simulink model "Backstep"  (Simulink 7.0)
settings: Solver=ode45  StartTime=0.0  StopTime=1000.0  RelTol=1e-3
undefined symbols (not defined in the file or in its folder): C_calc
libraries: marine_gnc x3, fordypningsprosjekt x1, simulink x1
settings Model: Creator=anderga  LastModifiedBy=anderga

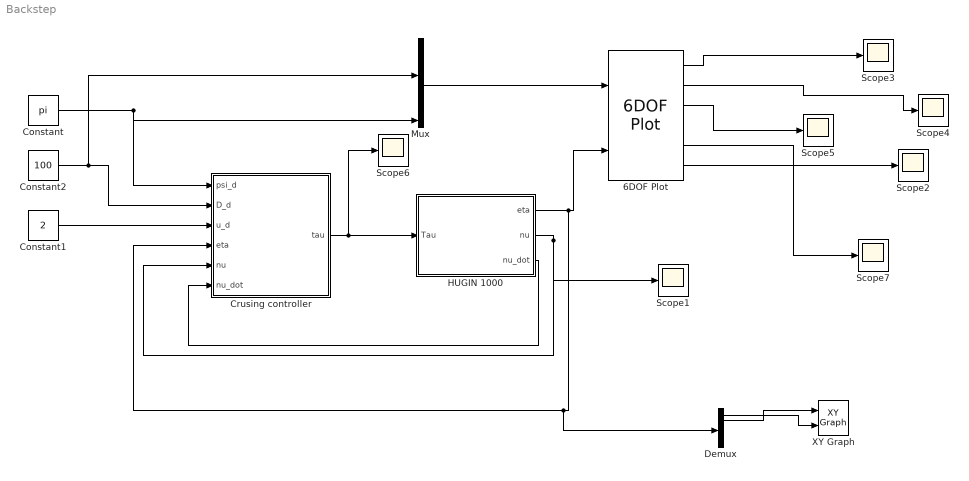
== system Backstep ==
  6DOF Plot : fordypningsprosjekt/6DOF Plot  SystemSampleTime=-1
  Constant : Constant  Value=pi  OutDataType=sfix(16)  OutScaling=2^0
  Constant1 : Constant  Value=2  OutDataType=sfix(16)  OutScaling=2^0
  Constant2 : Constant  Value=100  OutDataType=sfix(16)  OutScaling=2^0
  Crusing controller : Subsystem  mask{Kp_u=5, Ki_u=1, Kp_c=100, Kd_c=10, Kp_d=5, Kp2_d=2, Kd_d=4}
      mask prompts: Kp_u "Kp Speed controller"; Ki_u "Ki Speed Controller"; Kp_c "Kp Course Controller"; Kd_c "Kd Course Controller"; Kp_d "Kp1 Depth Controller"; Kp2_d "Kp2 Depth controller"; Kd_d "Kd Depth Controller"
  Demux : Demux  Outputs=6
  HUGIN 1000 : Subsystem  AncestorBlock=fordypningsprosjekt/HUGIN 1000  mask(HUGIN 1000 AUV){eta_0=[0 0 0 0 0 0], nu_0=[0 0 0 0 0 0]}
      mask prompts: eta_0 "Initial Position [x y z phi theta psi]"; nu_0 "Initial speed [u v w p q r]"
      mask help:
      | The hydrodynamic model of Kongsberg Maritimes
      | AUV type HUGIN 1000.
      |
      | Implemented using
      |
      | eta_dot = J(eta)*nu
      | M*nu_dot + C(nu)*nu + D(nu)*nu + g(eta) = tau
      |
      | and the MMS toolbox from www.marinecybernetics.org
      mask init:
      | m = 1380;
      | xg = 0;
      | yg = 0;
      | zg = 0.0328;
      | Ix = 86.53;
      | Iy = 1247;
      | Iz = 1247;
      | 
      | Xu = -85.57;
      | Yv = -1092.9;
      | Yr = -84.1448;
      | Zw = -1092.9;
      | Zq = 84.1448;
      | Mq = -795.1686;
      | Nr = -795.1686;
      |     
      | M = [m-Xu   0       0       0       m*zg    -m*yg;
      |      0      m-Yv    0       -m*zg   0       m*xg-Yr;
      |      0      0       m-Zw    m*yg    -m*xg-Zq 0;
      |      0      -m*zg   m*yg    Ix      0        0;
      |      m*zg   0       -m*xg-Zq 0      Iy-Mq    0;
      |      -m*yg  m*xg-Yr 0       0       0       Iz-Nr];
  Mux : Mux  Inputs=6
  Scope{1..7} (7 alike) : Scope
      Scope1 settings: YMin=-1  YMax=2.5
      Scope2 settings: TimeRange=1000  YMin=0  YMax=45
      Scope3 settings: TimeRange=1000  YMin=-1750  YMax=0  SaveName=ScopeData2
      Scope4 settings: YMin=0  YMax=275  SaveName=ScopeData3
      Scope5 settings: YMin=100  YMax=100  SaveName=ScopeData4
      Scope6 settings: YMax=55  SaveName=ScopeData5
      Scope7 settings: YMin=-90  YMax=70  SaveName=ScopeData6
  XY Graph : simulink/Sinks/XY Graph  SystemSampleTime=-1  xmin=-1000  xmax=1000  ymin=-1000  ymax=1000  st=-1
  wires:
  Crusing controller/1(tau) -> HUGIN 1000/1(Tau), Scope6/1
  HUGIN 1000/1(eta) -> 6DOF Plot/2, Crusing controller/4(eta), Demux/1
  HUGIN 1000/2(nu) -> Crusing controller/5(nu), Scope1/1
  HUGIN 1000/3(nu_dot) -> Crusing controller/6(nu_dot)
  Constant1/1 -> Crusing controller/3(u_d)
  Constant/1 -> Crusing controller/1(psi_d), Mux/6
  6DOF Plot/6 -> Scope2/1
  6DOF Plot/1 -> Scope3/1
  6DOF Plot/2 -> Scope4/1
  Mux/1 -> 6DOF Plot/1
  6DOF Plot/3 -> Scope5/1
  Constant2/1 -> Crusing controller/2(D_d), Mux/3
  6DOF Plot/5 -> Scope7/1
  Demux/2 -> XY Graph/1
  Demux/1 -> XY Graph/2

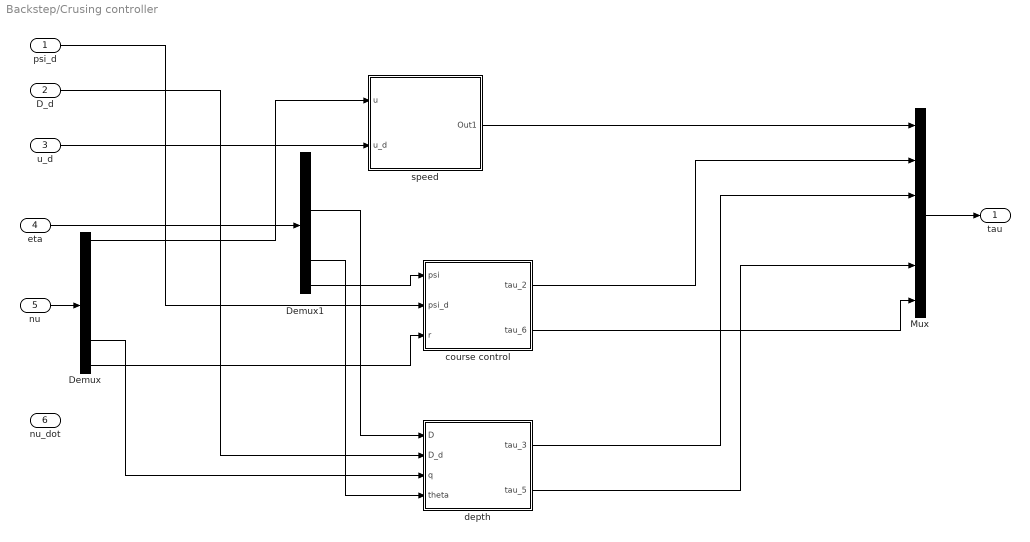
== system Backstep/Crusing controller ==
  psi_d : Inport  OutDataType=sfix(16)  OutScaling=2^0
  D_d : Inport  Port=2  OutDataType=sfix(16)  OutScaling=2^0
  u_d : Inport  Port=3  OutDataType=sfix(16)  OutScaling=2^0
  eta : Inport  Port=4  OutDataType=sfix(16)  OutScaling=2^0
  nu : Inport  Port=5  OutDataType=sfix(16)  OutScaling=2^0
  nu_dot : Inport  Port=6  OutDataType=sfix(16)  OutScaling=2^0
  Demux : Demux  Outputs=6
  Demux1 : Demux  Outputs=6
  Mux : Mux  Inputs=6
  course control : Subsystem
  depth : Subsystem
  speed : Subsystem
  tau : Outport  OutDataType=sfix(16)  OutScaling=2^0
  wires:
  nu/1 -> Demux/1
  Demux/1 -> speed/1(u)
  u_d/1 -> speed/2(u_d)
  eta/1 -> Demux1/1
  Demux1/6 -> course control/1(psi)
  psi_d/1 -> course control/2(psi_d)
  Demux/6 -> course control/3(r)
  speed/1(Out1) -> Mux/1
  Mux/1 -> tau/1
  course control/1(tau_2) -> Mux/2
  course control/2(tau_6) -> Mux/6
  D_d/1 -> depth/2(D_d)
  Demux1/3 -> depth/1(D)
  Demux/5 -> depth/3(q)
  Demux1/5 -> depth/4(theta)
  depth/1(tau_3) -> Mux/3
  depth/2(tau_5) -> Mux/5

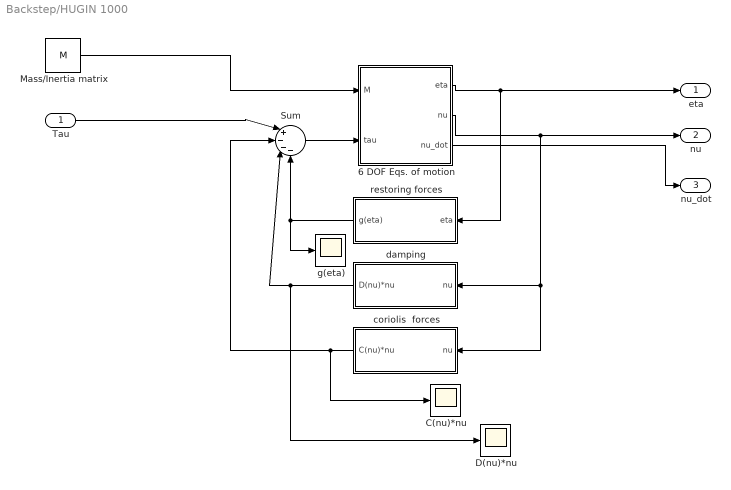
== system Backstep/HUGIN 1000 ==
  Tau : Inport  OutDataType=sfix(16)  OutScaling=2^0
  6 DOF Eqs. of motion : Subsystem  AncestorBlock=marine_gnc/Models/ Kinetics /6 DOF Eqs. of motion  mask(Equations of motion){nu0=nu_0, eta0=eta_0}
      mask prompts: nu0 "Initial velocities (u,v,w,p,q,r)"; eta0 "Initial position/attitude (x,y,z,phi,theta,psi)"
      mask help:
      | 6 DOF equations of motion (surge, sway, heave, roll, pitch and yaw)
      |
      |    eta_dot = J(eta)*nu
      |    (M_RB+M_A)*nu_dot  =  tau
      |
      | where nu = [u,v,w,p,q,r]'  and eta = [x,y,z,phi,theta,psi]'
      |
      | T. I. Fossen (2002). Marine Control Systems: Guidance, Navigation and Control of Ships, Rigs and Underwater Vehicles, Marine Cybernetics AS, ISBN 82-92356-00-2
      |
      | Modified by Anders Garmo (2008)
  C(nu)*nu : Scope
      settings: TimeRange=100  YMin=-0.1  YMax=1.2  SaveName=ScopeData5
  D(nu)*nu : Scope
      settings: TimeRange=100  YMin=-10  YMax=100  SaveName=ScopeData8
  Mass/Inertia matrix : Constant  Value=M  OutDataType=sfix(16)  OutScaling=2^0
  Sum : Sum  Inputs=|+---  OutDataType=sfix(16)  OutScaling=2^0
  coriolis  forces : Subsystem  Orientation=left
      mask init:
      | W = 1380*9.81;
      | 
      | zg = 0.0328;
  damping : Subsystem  Orientation=left
      mask init:
      | Xu = -19.1881;
      | Yv = -931.9715;
      | Yr = 1915.8;
      | Zw = -931.9715;
      | Zq = -1915.8;
      | Kp = -1000;
      | Mw = 1760.7;
      | Mq = -8386.3;
      | Nv = -1760.7;
      | Nr = -8386.3;
      | 
      | Xuu = -3.8938;
      | 
      | D = [Xu 0 0 0 0 0;
      |       0 Yv 0 0 0 Yr;
      |       0 0 Zw 0 Zq 0;
      |       0 0 0 Kp 0 0;
      |       0 0 Mw 0 Mq 0;
      |       0 Nv 0 0 0 Nr];
  g(eta) : Scope
      settings: TimeRange=100  YMin=0  YMax=100  SaveName=ScopeData7
  restoring forces : Subsystem  Orientation=left
      mask init:
      | W = 1380*9.81;
      | 
      | zg = 0.0328;
  eta : Outport  OutDataType=sfix(16)  OutScaling=2^0
  nu : Outport  Port=2  OutDataType=sfix(16)  OutScaling=2^0
  nu_dot : Outport  Port=3  OutDataType=sfix(16)  OutScaling=2^0
  wires:
  Mass/Inertia matrix/1 -> 6 DOF Eqs. of motion/1(M)
  6 DOF Eqs. of motion/2(nu) -> nu/1, damping/1(nu), coriolis  forces/1(nu)
  6 DOF Eqs. of motion/1(eta) -> restoring forces/1(eta), eta/1
  Sum/1 -> 6 DOF Eqs. of motion/2(tau)
  Tau/1 -> Sum/1
  coriolis  forces/1(C(nu)*nu) -> C(nu)*nu/1, Sum/2
  restoring forces/1(g(eta)) -> Sum/4, g(eta)/1
  damping/1(D(nu)*nu) -> Sum/3, D(nu)*nu/1
  6 DOF Eqs. of motion/3(nu_dot) -> nu_dot/1

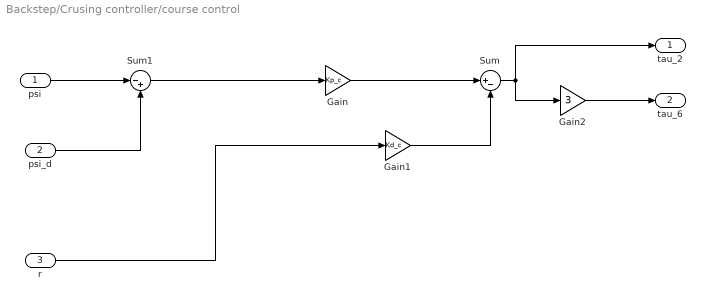
== system Backstep/Crusing controller/course control ==
  psi : Inport  OutDataType=sfix(16)  OutScaling=2^0
  psi_d : Inport  Port=2  OutDataType=sfix(16)  OutScaling=2^0
  r : Inport  Port=3  OutDataType=sfix(16)  OutScaling=2^0
  Gain : Gain  Gain=Kp_c  ParameterDataType=sfix(16)  ParameterScaling=2^0  OutDataType=sfix(16)  OutScaling=2^0
  Gain1 : Gain  Gain=Kd_c  ParameterDataType=sfix(16)  ParameterScaling=2^0  OutDataType=sfix(16)  OutScaling=2^0
  Gain2 : Gain  Gain=3  ParameterDataType=sfix(16)  ParameterScaling=2^0  OutDataType=sfix(16)  OutScaling=2^0
  Sum : Sum  Inputs=|+-  OutDataType=sfix(16)  OutScaling=2^0
  Sum1 : Sum  Inputs=|-+  OutDataType=sfix(16)  OutScaling=2^0
  tau_2 : Outport  OutDataType=sfix(16)  OutScaling=2^0
  tau_6 : Outport  Port=2  OutDataType=sfix(16)  OutScaling=2^0
  wires:
  Sum1/1 -> Gain/1
  Gain1/1 -> Sum/2
  psi/1 -> Sum1/1
  psi_d/1 -> Sum1/2
  Gain/1 -> Sum/1
  r/1 -> Gain1/1
  Sum/1 -> Gain2/1, tau_2/1
  Gain2/1 -> tau_6/1

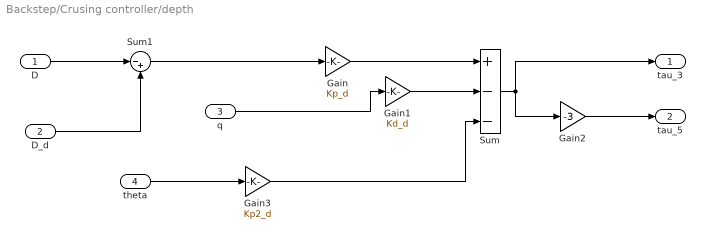
== system Backstep/Crusing controller/depth ==
  D : Inport  OutDataType=sfix(16)  OutScaling=2^0
  D_d : Inport  Port=2  OutDataType=sfix(16)  OutScaling=2^0
  q : Inport  Port=3  OutDataType=sfix(16)  OutScaling=2^0
  theta : Inport  Port=4  OutDataType=sfix(16)  OutScaling=2^0
  Gain : Gain  Gain=Kp_d  ParameterDataType=sfix(16)  ParameterScaling=2^0  OutDataType=sfix(16)  OutScaling=2^0
  Gain1 : Gain  Gain=Kd_d  ParameterDataType=sfix(16)  ParameterScaling=2^0  OutDataType=sfix(16)  OutScaling=2^0
  Gain2 : Gain  Gain=-3  ParameterDataType=sfix(16)  ParameterScaling=2^0  OutDataType=sfix(16)  OutScaling=2^0
  Gain3 : Gain  Gain=Kp2_d  ParameterDataType=sfix(16)  ParameterScaling=2^0  OutDataType=sfix(16)  OutScaling=2^0
  Sum : Sum  Inputs=+--  OutDataType=sfix(16)  OutScaling=2^0
  Sum1 : Sum  Inputs=|-+  OutDataType=sfix(16)  OutScaling=2^0
  tau_3 : Outport  OutDataType=sfix(16)  OutScaling=2^0
  tau_5 : Outport  Port=2  OutDataType=sfix(16)  OutScaling=2^0
  wires:
  Gain2/1 -> tau_5/1
  Sum/1 -> tau_3/1, Gain2/1
  q/1 -> Gain1/1
  Gain/1 -> Sum/1
  D_d/1 -> Sum1/2
  D/1 -> Sum1/1
  Gain1/1 -> Sum/2
  Sum1/1 -> Gain/1
  theta/1 -> Gain3/1
  Gain3/1 -> Sum/3

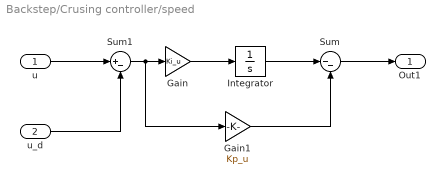
== system Backstep/Crusing controller/speed ==
  u : Inport  OutDataType=sfix(16)  OutScaling=2^0
  u_d : Inport  Port=2  OutDataType=sfix(16)  OutScaling=2^0
  Gain : Gain  Gain=Ki_u  ParameterDataType=sfix(16)  ParameterScaling=2^0  OutDataType=sfix(16)  OutScaling=2^0
  Gain1 : Gain  Gain=Kp_u  ParameterDataType=sfix(16)  ParameterScaling=2^0  OutDataType=sfix(16)  OutScaling=2^0
  Integrator : Integrator
  Sum : Sum  Inputs=|--  OutDataType=sfix(16)  OutScaling=2^0
  Sum1 : Sum  Inputs=|+-  OutDataType=sfix(16)  OutScaling=2^0
  Out1 : Outport  OutDataType=sfix(16)  OutScaling=2^0
  wires:
  Sum/1 -> Out1/1
  u/1 -> Sum1/1
  u_d/1 -> Sum1/2
  Sum1/1 -> Gain/1, Gain1/1
  Integrator/1 -> Sum/1
  Gain/1 -> Integrator/1
  Gain1/1 -> Sum/2

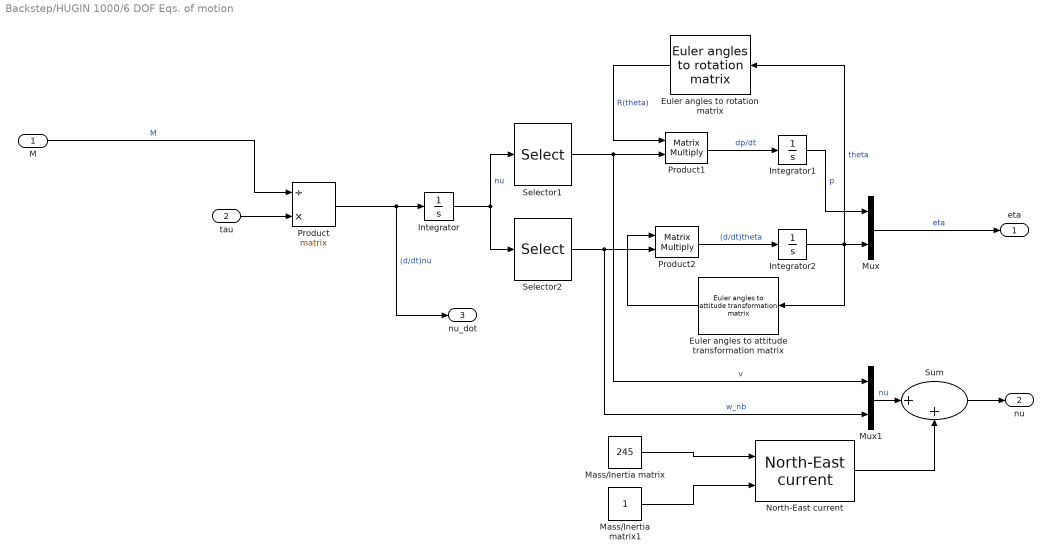
== system Backstep/HUGIN 1000/6 DOF Eqs. of motion ==
  M : Inport  OutDataType=sfix(16)  OutScaling=2^0
  tau : Inport  Port=2  OutDataType=sfix(16)  OutScaling=2^0
  Euler angles to rotation matrix : marine_gnc/Models/ Kinematics/Euler angles to rotation matrix  Orientation=left  SystemSampleTime=-1
  Euler angles to attitude transformation matrix : marine_gnc/Models/ Kinematics/Euler angles to attitude transformation matrix  Orientation=left  SystemSampleTime=-1
  Integrator : Integrator  InitialCondition=nu0
  Integrator1 : Integrator  InitialCondition=eta0(1:3)
  Integrator2 : Integrator  InitialCondition=eta0(4:6)
  Mass/Inertia matrix : Constant  Value=245  OutDataType=sfix(16)  OutScaling=2^0
  Mass/Inertia matrix1 : Constant  OutDataType=sfix(16)  OutScaling=2^0
  Mux : Mux  Inputs=2
  Mux1 : Mux  Inputs=2
  North-East current : marine_gnc/Environment/Current/North-East current  SystemSampleTime=-1
  Product : Product  Inputs=/*  Multiplication=Matrix(*)  OutDataType=sfix(16)  OutScaling=2^0  SaturateOnIntegerOverflow=on
  Product1 : Product  Inputs=**  Multiplication=Matrix(*)  OutDataType=sfix(16)  OutScaling=2^0  SaturateOnIntegerOverflow=on
  Product2 : Product  Inputs=**  Multiplication=Matrix(*)  OutDataType=sfix(16)  OutScaling=2^0  SaturateOnIntegerOverflow=on
  Selector1 : Selector  InputPortWidth=6  IndexOptions=Index vector (dialog)  Indices=[1 2 3]  OutputSizes=1
  Selector2 : Selector  InputPortWidth=6  IndexOptions=Index vector (dialog)  Indices=[4 5 6]  OutputSizes=1
  Sum : Sum  Inputs=|++  OutDataType=sfix(16)  OutScaling=2^0
  eta : Outport  OutDataType=sfix(16)  OutScaling=2^0
  nu : Outport  Port=2  OutDataType=sfix(16)  OutScaling=2^0
  nu_dot : Outport  Port=3  OutDataType=sfix(16)  OutScaling=2^0
  wires:
  tau/1 -> Product/2
  Euler angles to attitude transformation matrix/1 -> Product2/1
  Mux/1 -> eta/1  "eta"
  Integrator1/1 -> Mux/1  "p"
  Integrator2/1 -> Euler angles to attitude transformation matrix/1, Euler angles to rotation matrix/1, Mux/2  "theta"
  Product2/1 -> Integrator2/1  "(d/dt)theta"
  Euler angles to rotation matrix/1 -> Product1/1  "R(theta)"
  Product1/1 -> Integrator1/1  "dp/dt"
  Selector2/1 -> Product2/2, Mux1/2  "w_nb"
  Selector1/1 -> Mux1/1, Product1/2  "v"
  Integrator/1 -> Selector2/1, Selector1/1  "nu"
  Product/1 -> Integrator/1, nu_dot/1  "(d/dt)nu"
  M/1 -> Product/1  "M"
  Mux1/1 -> Sum/1  "nu"
  Sum/1 -> nu/1
  North-East current/1 -> Sum/2
  Mass/Inertia matrix/1 -> North-East current/1
  Mass/Inertia matrix1/1 -> North-East current/2

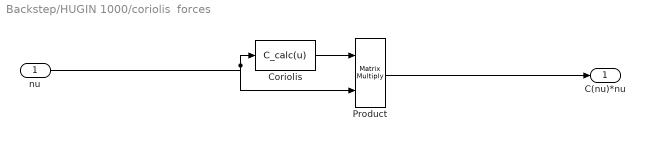
== system Backstep/HUGIN 1000/coriolis  forces ==
  nu : Inport  OutDataType=sfix(16)  OutScaling=2^0
  Coriolis : MATLABFcn  MATLABFcn=C_calc(u)  OutputDimensions=[6,6]  Output1D=off
  Product : Product  Multiplication=Matrix(*)  OutDataType=sfix(16)  OutScaling=2^0  RndMeth=Zero
  C(nu)*nu : Outport  OutDataType=sfix(16)  OutScaling=2^0
  wires:
  nu/1 -> Product/2, Coriolis/1
  Coriolis/1 -> Product/1
  Product/1 -> C(nu)*nu/1

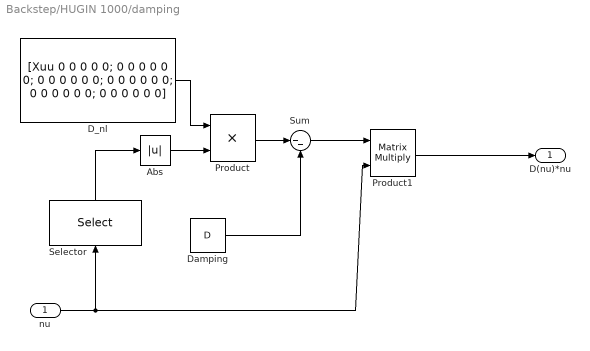
== system Backstep/HUGIN 1000/damping ==
  nu : Inport  OutDataType=sfix(16)  OutScaling=2^0
  Abs : Abs  OutDataType=sfix(16)  OutScaling=2^0
  D_nl : Constant  Value=[Xuu 0 0 0 0 0; 0 0 0 0 0 0; 0 0 0 0 0 0; 0 0 0 0 0 0; 0 0 0 0 0 0; 0 0 0 0 0 0]  OutDataType=sfix(16)  OutScaling=2^0
  Damping : Constant  Value=D  OutDataType=sfix(16)  OutScaling=2^0
  Product : Product  OutDataType=sfix(16)  OutScaling=2^0  RndMeth=Zero
  Product1 : Product  Multiplication=Matrix(*)  OutDataType=sfix(16)  OutScaling=2^0  RndMeth=Zero
  Selector : Selector  Orientation=up  InputPortWidth=6  IndexOptions=Index vector (dialog)  Indices=[1]  OutputSizes=1
  Sum : Sum  Inputs=|--  OutDataType=sfix(16)  OutScaling=2^0
  D(nu)*nu : Outport  OutDataType=sfix(16)  OutScaling=2^0
  wires:
  Damping/1 -> Sum/2
  Product/1 -> Sum/1
  nu/1 -> Product1/2, Selector/1
  D_nl/1 -> Product/1
  Abs/1 -> Product/2
  Sum/1 -> Product1/1
  Product1/1 -> D(nu)*nu/1
  Selector/1 -> Abs/1

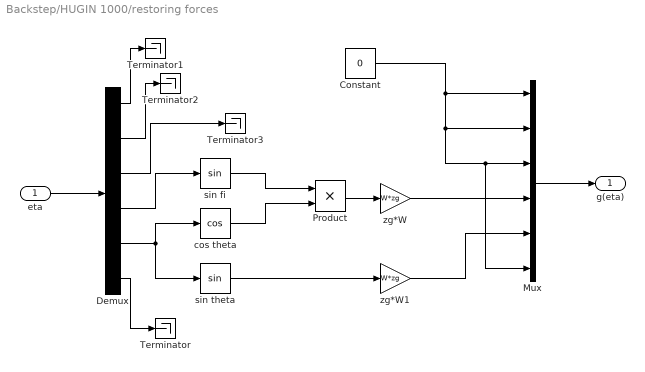
== system Backstep/HUGIN 1000/restoring forces ==
  eta : Inport  OutDataType=sfix(16)  OutScaling=2^0
  Constant : Constant  Value=0  OutDataType=sfix(16)  OutScaling=2^0
  Demux : Demux  Outputs=6
  Mux : Mux  Inputs=6
  Product : Product  OutDataType=sfix(16)  OutScaling=2^0  RndMeth=Zero
  Terminator{,1..3} (4 alike) : Terminator
  cos theta : Trigonometry  Operator=cos
  sin fi : Trigonometry
  sin theta : Trigonometry
  zg*W : Gain  Gain=W*zg  ParameterDataType=sfix(16)  ParameterScaling=2^0  OutDataType=sfix(16)  OutScaling=2^0
  zg*W1 : Gain  Gain=W*zg  ParameterDataType=sfix(16)  ParameterScaling=2^0  OutDataType=sfix(16)  OutScaling=2^0
  g(eta) : Outport  OutDataType=sfix(16)  OutScaling=2^0
  wires:
  eta/1 -> Demux/1
  Demux/4 -> sin fi/1
  Demux/5 -> cos theta/1, sin theta/1
  cos theta/1 -> Product/2
  sin fi/1 -> Product/1
  Product/1 -> zg*W/1
  sin theta/1 -> zg*W1/1
  Mux/1 -> g(eta)/1
  zg*W1/1 -> Mux/5
  zg*W/1 -> Mux/4
  Constant/1 -> Mux/1, Mux/2, Mux/3, Mux/6
  Demux/6 -> Terminator/1
  Demux/1 -> Terminator1/1
  Demux/2 -> Terminator2/1
  Demux/3 -> Terminator3/1
